simulink model "DSCA_testing"  (R2016b)
settings: Solver=FixedStepDiscrete  StartTime=0.0  StopTime=10.0  FixedStep=CAL_EncoderSampleTime  RelTol=1e-3
undefined symbols (not defined in the file): sigbuilder_block
libraries: DSCA x1
settings Model: Creator=oelkawok  LastModifiedBy=oelkawok

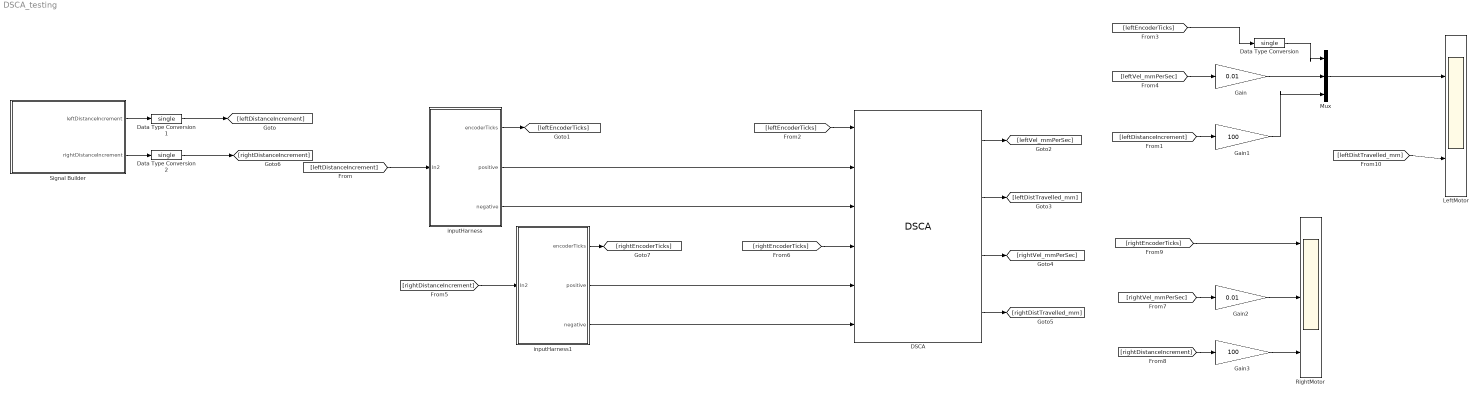
== system DSCA_testing ==
  DSCA : DSCA/DSCA
  Data Type Conversion : DataTypeConversion  OutDataTypeStr=single
  Data Type Conversion1 : DataTypeConversion  OutDataTypeStr=single
  Data Type Conversion2 : DataTypeConversion  OutDataTypeStr=single
  Gain : Gain  Gain=0.01
  Gain1 : Gain  Gain=100
  Gain2 : Gain  Gain=0.01
  Gain3 : Gain  Gain=100
  LeftMotor : Scope  NumInputPorts=2
  Mux : Mux  Inputs=3
  RightMotor : Scope  NumInputPorts=3
  Signal Builder : Subsystem  Tag=STV Subsys  LoadFcn=sigbuilder_block('load');  StartFcn=sigbuilder_block('start');  StopFcn=sigbuilder_block('stop');  ClipboardFcn=sigbuilder_block('clipboard');  mask(Sigbuilder block){tuvar=[0:10]}
      mask help: Simulink:masks:SigbuilderBlock_MD
      mask init:
      | if ~strcmp(get_param(bdroot(gcbh),'SimulationStatus'),'stopped') tuvar = sigbuilder_block('maskInit'); end
      settings: CopyFcn=sigbuilder_block('copy');  DeleteFcn=sigbuilder_block('delete');  ModelCloseFcn=sigbuilder_block('modelClose');  PreSaveFcn=sigbuilder_block('preSave');  PauseFcn=sigbuilder_block('pause');  ContinueFcn=sigbuilder_block('continue');  NameChangeFcn=sigbuilder_block('namechange');  OpenFcn=sigbuilder_block('open',[0.6 30.6 574.8 555.6 ]);  CloseFcn=sigbuilder_block('close');
      mask Display: plot(0, 0, 100, 100,[2, 2, 32, 32, 2], [68, 8, 8, 68, 68],[32, 2], [38, 38], [32, 19, 2],[53, 60, 44], [32, 17, 17, 2],[16, 16, 31, 31]);txt = getActiveGroup(gcbh);text(2, 100, txt,'verticalAlignment', 'top');
  inputHarness : Subsystem
  inputHarness1 : Subsystem
  wires:
  inputHarness/2(positive) -> DSCA/2
  inputHarness/3(negative) -> DSCA/3
  Signal Builder/1(leftDistanceIncrement) -> Data Type Conversion1/1
  [leftDistanceIncrement] -> inputHarness/1(In2)
  [leftDistanceIncrement] -> Gain1/1
  inputHarness/1(encoderTicks) -> [leftEncoderTicks]
  [leftEncoderTicks] -> DSCA/1
  DSCA/1 -> [leftVel_mmPerSec]
  [leftVel_mmPerSec] -> Gain/1
  DSCA/2 -> [leftDistTravelled_mm]
  DSCA/3 -> [rightVel_mmPerSec]
  DSCA/4 -> [rightDistTravelled_mm]
  Signal Builder/2(rightDistanceIncrement) -> Data Type Conversion2/1
  [rightDistanceIncrement] -> inputHarness1/1(In2)
  inputHarness1/2(positive) -> DSCA/5
  inputHarness1/3(negative) -> DSCA/6
  inputHarness1/1(encoderTicks) -> [rightEncoderTicks]
  [rightEncoderTicks] -> DSCA/4
  Gain2/1 -> RightMotor/2
  Gain3/1 -> RightMotor/3
  [rightEncoderTicks] -> RightMotor/1
  [rightVel_mmPerSec] -> Gain2/1
  [rightDistanceIncrement] -> Gain3/1
  Gain1/1 -> Mux/3
  Gain/1 -> Mux/2
  [leftEncoderTicks] -> Data Type Conversion/1
  Mux/1 -> LeftMotor/1
  [leftDistTravelled_mm] -> LeftMotor/2
  Data Type Conversion1/1 -> [leftDistanceIncrement]
  Data Type Conversion2/1 -> [rightDistanceIncrement]
  Data Type Conversion/1 -> Mux/1

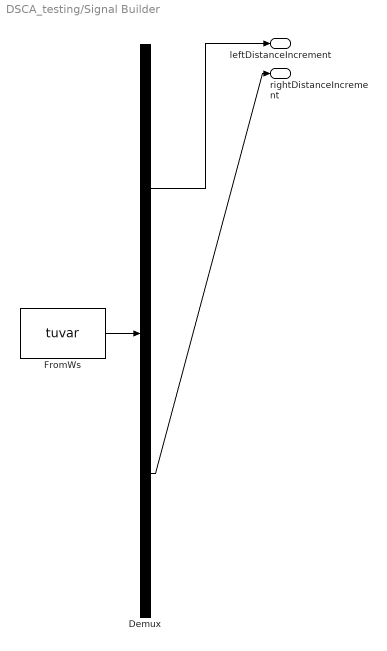
== system DSCA_testing/Signal Builder ==
  Demux : Demux  Tag=STV Demux  Outputs=2
  FromWs : FromWorkspace  Tag=STV FromWs  VariableName=tuvar  SampleTime=0
      SigBuilderData=|
      | common.afterFinalStr = 'Extrapolate'
      | common.sampleTime = 0
      | dataSet(1).timeRange = [0 10]
      | dataSet(1).name = 'Group 1'
      | dataSet(2).timeRange = [0 10]
      | dataSet(2).name = 'Group 2'
      | sbobj.Groups(1).Name = 'Group 1'
      | sbobj.Groups(1).Signals(1).Name = 'leftDistanceIncrement'
      | sbobj.Groups(1).Signals(1).XData = [0 1.9 3.98 4.94 6.2 7 8.2 8.76 10]
      | sbobj.Groups(1).Signals(1).YData = [0 0.00134 0 0.01 0.0008 0 0 0.001 0]
      | sbobj.Groups(1).Signals(2).Name = 'rightDistanceIncrement'
      | sbobj.Groups(1).Signals(2).XData = [0 1.9 3.98 4.94 6.2 7 8.2 8.76 10]
      | sbobj.Groups(1).Signals(2).YData = [0 0.00134 0 0.01 0.0008 0 0 0.001 0]
      | sbobj.Groups(2).Name = 'Group 2'
      | sbobj.Groups(2).Signals(1).Name = 'leftDistanceIncrement'
      | sbobj.Groups(2).Signals(1).XData = [0 1.9 3 4.94 6 7 8.2 8.76 9.02 10]
      | sbobj.Groups(2).Signals(1).YData = [0 0.00134 0.015 0.015 -0.01 -0.01 0.01 0.01 0 0]
      | sbobj.Groups(2).Signals(2).Name = 'rightDistanceIncrement'
      | sbobj.Groups(2).Signals(2).XData = [0 1.9 3 4.94 6 7 8.2 8.76 9.02 10]
      | sbobj.Groups(2).Signals(2).YData = [0 0.00134 0.015 0.015 -0.01 -0.01 0.01 0.01 0 0]
  leftDistanceIncrement : Outport  Tag=STV Outport
  rightDistanceIncrement : Outport  Tag=STV Outport  Port=2
  wires:
  Demux/1 -> leftDistanceIncrement/1
  FromWs/1 -> Demux/1
  Demux/2 -> rightDistanceIncrement/1

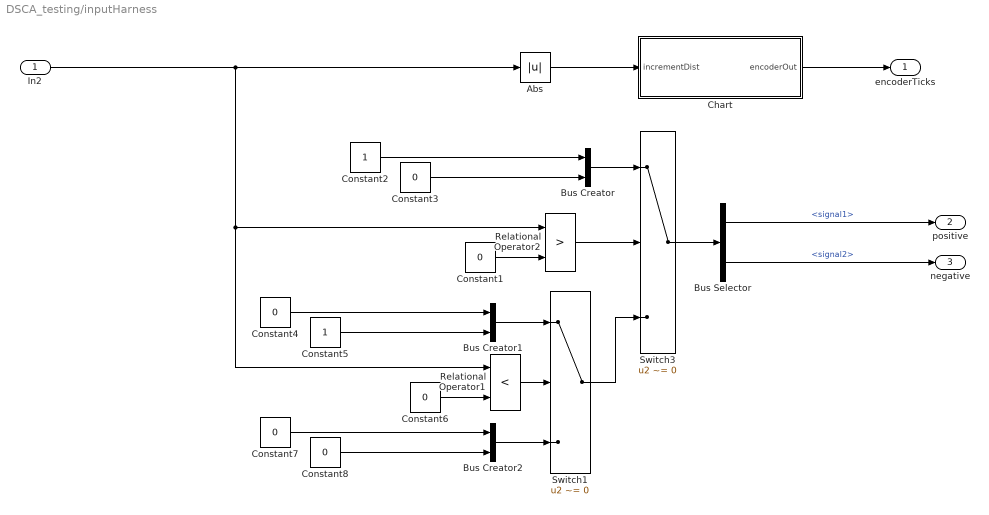
== system DSCA_testing/inputHarness ==
  In2 : Inport
  Abs : Abs
  Bus Creator : BusCreator  Inputs=2
  Bus Creator1 : BusCreator  Inputs=2
  Bus Creator2 : BusCreator  Inputs=2
  Bus Selector : BusSelector  OutputSignals=signal1,signal2
  Chart : Stateflow chart  TreatAsAtomicUnit=on
  Constant{1,3..4,6..8} (6 alike) : Constant  Value=0
  Constant2 : Constant
  Constant5 : Constant
  Relational Operator1 : RelationalOperator  Operator=<  OutDataTypeStr=boolean  RndMeth=Simplest
  Relational Operator2 : RelationalOperator  Operator=>  OutDataTypeStr=boolean  RndMeth=Simplest
  Switch1 : Switch  Criteria=u2 ~= 0
  Switch3 : Switch  Criteria=u2 ~= 0
  encoderTicks : Outport
  positive : Outport  Port=2
  negative : Outport  Port=3
  wires:
  In2/1 -> Relational Operator2/1, Relational Operator1/1, Abs/1
  Constant2/1 -> Bus Creator/1
  Constant8/1 -> Bus Creator2/2
  Bus Selector/1 -> positive/1  "<signal1>"
  Constant3/1 -> Bus Creator/2
  Bus Selector/2 -> negative/1  "<signal2>"
  Constant4/1 -> Bus Creator1/1
  Bus Creator1/1 -> Switch1/1
  Bus Creator/1 -> Switch3/1
  Chart/1(encoderOut) -> encoderTicks/1
  Relational Operator1/1 -> Switch1/2
  Relational Operator2/1 -> Switch3/2
  Constant7/1 -> Bus Creator2/1
  Bus Creator2/1 -> Switch1/3
  Switch3/1 -> Bus Selector/1
  Constant1/1 -> Relational Operator2/2
  Abs/1 -> Chart/1(incrementDist)
  Switch1/1 -> Switch3/3
  Constant5/1 -> Bus Creator1/2
  Constant6/1 -> Relational Operator1/2

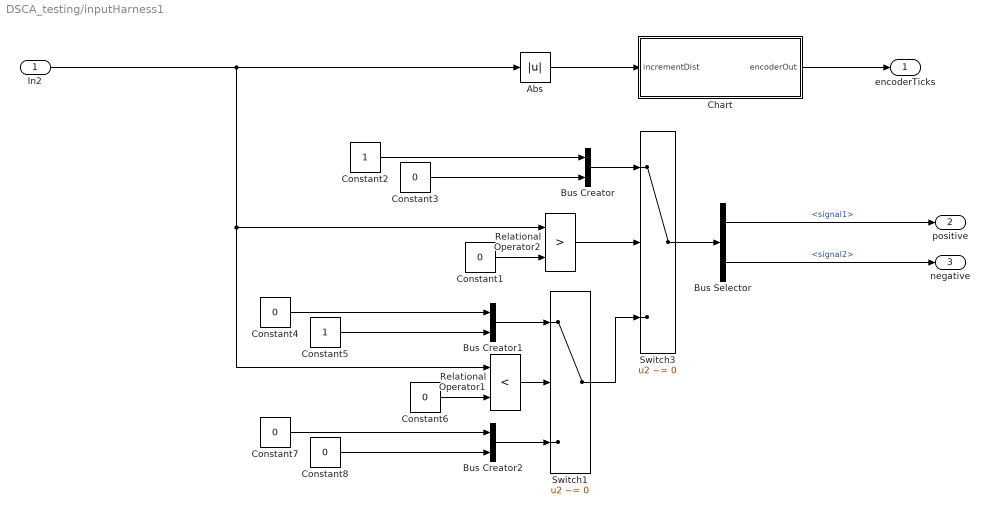
== system DSCA_testing/inputHarness1 ==
  In2 : Inport
  Abs : Abs
  Bus Creator : BusCreator  Inputs=2
  Bus Creator1 : BusCreator  Inputs=2
  Bus Creator2 : BusCreator  Inputs=2
  Bus Selector : BusSelector  OutputSignals=signal1,signal2
  Chart : Stateflow chart  TreatAsAtomicUnit=on
  Constant{1,3..4,6..8} (6 alike) : Constant  Value=0
  Constant2 : Constant
  Constant5 : Constant
  Relational Operator1 : RelationalOperator  Operator=<  OutDataTypeStr=boolean  RndMeth=Simplest
  Relational Operator2 : RelationalOperator  Operator=>  OutDataTypeStr=boolean  RndMeth=Simplest
  Switch1 : Switch  Criteria=u2 ~= 0
  Switch3 : Switch  Criteria=u2 ~= 0
  encoderTicks : Outport
  positive : Outport  Port=2
  negative : Outport  Port=3
  wires:
  Constant6/1 -> Relational Operator1/2
  Constant5/1 -> Bus Creator1/2
  Switch1/1 -> Switch3/3
  Abs/1 -> Chart/1(incrementDist)
  Constant1/1 -> Relational Operator2/2
  Switch3/1 -> Bus Selector/1
  Bus Creator2/1 -> Switch1/3
  Constant7/1 -> Bus Creator2/1
  Relational Operator2/1 -> Switch3/2
  Relational Operator1/1 -> Switch1/2
  Chart/1(encoderOut) -> encoderTicks/1
  Bus Creator/1 -> Switch3/1
  Bus Creator1/1 -> Switch1/1
  Constant4/1 -> Bus Creator1/1
  Bus Selector/2 -> negative/1  "<signal2>"
  Constant3/1 -> Bus Creator/2
  Bus Selector/1 -> positive/1  "<signal1>"
  Constant8/1 -> Bus Creator2/2
  Constant2/1 -> Bus Creator/1
  In2/1 -> Abs/1, Relational Operator1/1, Relational Operator2/1

== stateflow chart DSCA_testing/inputHarness1/Chart ==
  (default) -> (junction 1) : {
      | localDist = localDist + incrementDist;
      | }
  (junction 1) -> (junction 3) [order 1] : [localDist >= 0.036]//0.026]
  (junction 1) -> (junction 11) [order 2]
  (junction 3) -> (junction 5) : {
      | encoderOut = true;
      | localDist = 0;
      | }
  (junction 11) -> (junction 13) [order 1] : [localDist >= 0.018]//0.013]
  (junction 13) -> (junction 15) : {
      | encoderOut = false;
      | }
  (junction 11) -> (junction 18) [order 2]
  (junction 15) -> (junction 18)
  (junction 5) -> (junction 15)
  data: encoderOut output boolean; incrementDist input; localDist local double

== stateflow chart DSCA_testing/inputHarness/Chart ==
  (default) -> (junction 1) : {
      | localDist = localDist + incrementDist;
      | }
  (junction 1) -> (junction 3) [order 1] : [localDist >= 0.036]//0.026]
  (junction 1) -> (junction 11) [order 2]
  (junction 3) -> (junction 5) : {
      | encoderOut = true;
      | localDist = 0;
      | }
  (junction 11) -> (junction 13) [order 1] : [localDist >= 0.018]//0.013]
  (junction 13) -> (junction 15) : {
      | encoderOut = false;
      | }
  (junction 11) -> (junction 18) [order 2]
  (junction 15) -> (junction 18)
  (junction 5) -> (junction 15)
  data: encoderOut output boolean; incrementDist input; localDist local double
